simulink model "tire2model"  (R2024b)
settings: Solver=VariableStepAuto  StartTime=0.0  StopTime=20  RelTol=1e-3
PreLoadFcn:
  | Tire = coder.load('Hoosier_R25B_16x75-10x7.mat', 'Tire');
values from neighbouring files (symbols this model uses):
  drive_train_eff = 0.95    [constants.mat]    (also in vehcileConstants2025.m)
  g = 9.81    [constants.mat]    (also in vehcileConstants2025.m)
  i_g = 2.91    [constants.mat]    (also in vehcileConstants2025.m)
  Idx = 1    [ContactPatchLoads.m]    (also in TireEvalModel.m; constants.mat; testing.m; vehcileConstants2025.m)
  Inclination = Inclination   .* (-1).^(mod(Idx+1,2))    [ContactPatchLoads.m]    (also in TireEvalModel.m = params.Inclination; constants.mat = 1; testing.m = 1; vehcileConstants2025.m = 1)
  lr = 0.859026    [constants.mat]    (also in vehcileConstants2025.m)
  m =     [constants.mat]
  Pressure = 70    [ContactPatchLoads.m]    (also in TireEvalModel.m = params.Pressure; constants.mat; testing.m; vehcileConstants2025.m)
  torque_vs_RPM_breakpoints = [0 5500 6048 6500]    [constants.mat]    (also in vehcileConstants2025.m = [0, 5500, 6048, 6500])
  torque_vs_RPM_table = [220 220 170 0]    [constants.mat]    (also in vehcileConstants2025.m = [220, 220, 170, 0])
  wheel =     [constants.mat]
libraries: slpidlib x1, autolibshared x1
settings Model: Creator=nhola  LastModifiedBy=nhola
settings DataIOCC: ExternalInput=[Model Tire]  LoadExternalInput=on
settings DebuggingCC: UnderSpecifiedDimensionMsg=warning

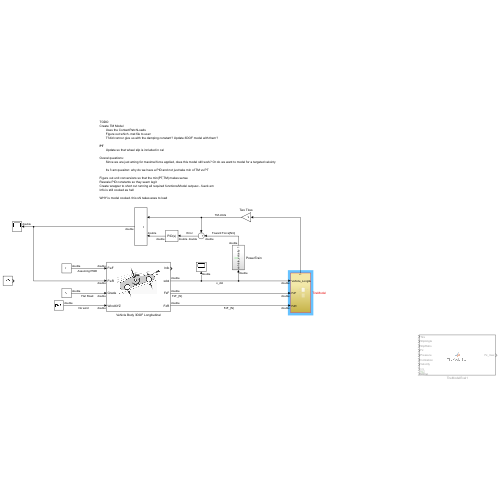
[thumbnail: Simulink's stored preview of the top-level diagram]
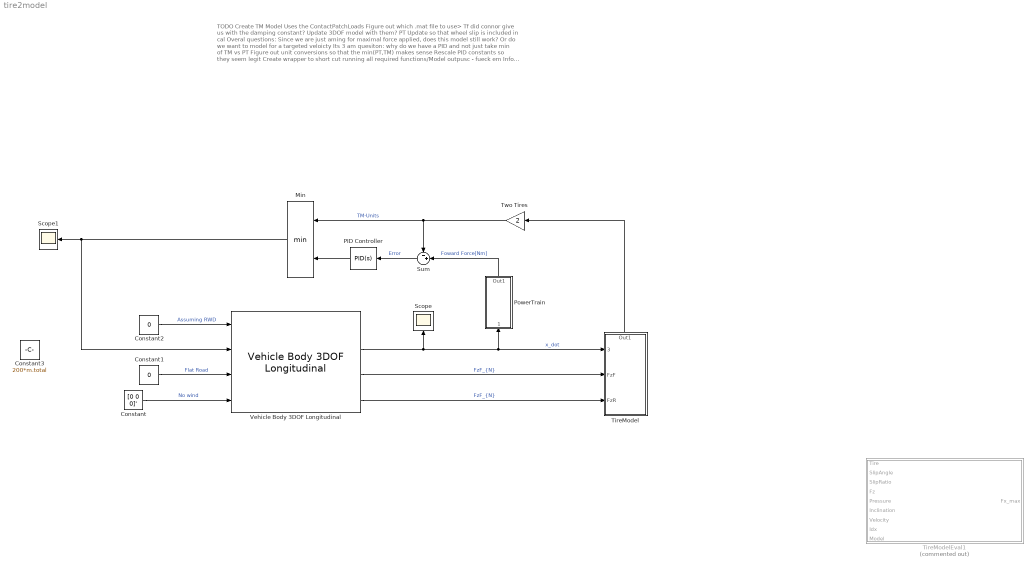
== system tire2model ==
  note: TODO
      | Create TM Model
      | Uses the ContactPatchLoads
      | Figure out which .mat file to use>
      | Tf did connor give us with the damping constant? Update 3DOF model with them?
      |
      | PT
      | Update so that wheel slip is included in cal
      |
      | Overal questions:
      | Since we are just aming for maximal force applied, does this model still work? Or do we want to model for a targeted veloicty
      |
      | Its 3 am quesiton: why do we have a PID and not just take min of TM vs PT
      |
      | Figure out unit conversions so that the min(PT,TM) makes sense
      | Rescale PID constants so they seem legit
      | Create wrapper to short cut running all required functions/Model outpusc - fueck em
      | Info is still cooked as hell
      |
      | WHY is model cooked, this shi takes ages to load
  Constant : Constant  Value=[0 0 0]'  VectorParams1D=off
  Constant1 : Constant  Value=0
  Constant2 : Constant  Value=0
  Constant3 : Constant  Value=200*m.total
  Min : MinMax  Inputs=2
  PID Controller : slpidlib/PID Controller  Controller=PID  Form=Parallel  TimeDomain=Continuous-time  UseExternalTs=off  SampleTime=-1  IntegratorMethod=Forward Euler  FilterMethod=Forward Euler  ControllerParametersSource=internal  P=m.total/5  I=m.total/25  UseKiTs=off  D=m.total/10  UseExternalDerivativeSource=off  N=100  UseFilter=on  TunerSelectOption=Transfer Function Based (PID Tuner App)  InitialConditionSource=internal  InitialConditionForIntegrator=0  InitialConditionForFilter=0  DifferentiatorICPrevScaledInput=0  ExternalReset=none  TrackingMode=off  Kt=1  LimitOutput=off  SatLimitsSource=internal  UpperSaturationLimit=inf  LowerSaturationLimit=-inf  LinearizeAsGain=on  AntiWindupMode=none  Kb=1  LimitIntegrator=off  UpperIntegratorSaturationLimit=inf  LowerIntegratorSaturationLimit=-inf  POutMin=[]  POutMax=[]  IOutMin=[]  IOutMax=[]  DOutMin=[]  DOutMax=[]  NOutMin=[]  NOutMax=[]  SumOutMin=[]  SumOutMax=[]  SaturationOutMin=[]  SaturationOutMax=[]  PParamMin=[]  PParamMax=[]  IParamMin=[]  IParamMax=[]  DParamMin=[]  DParamMax=[]  NParamMin=[]  NParamMax=[]  KbParamMin=[]  KbParamMax=[]  KtParamMin=[]  KtParamMax=[]  KbOutMin=[]  KbOutMax=[]  KtOutMin=[]  KtOutMax=[]  IntegratorOutMin=[]  IntegratorOutMax=[]  FilterOutMin=[]  FilterOutMax=[]  SumI1OutMin=[]  SumI1OutMax=[]  SumI2OutMin=[]  SumI2OutMax=[]  SumI3OutMin=[]  SumI3OutMax=[]  SumI4OutMin=[]  SumI4OutMax=[]  SumDOutMin=[]  SumDOutMax=[]  DifferentiatorOutMin=[]  DifferentiatorOutMax=[]  FilterDiffOutCoefMin=[]  FilterDiffOutCoefMax=[]  ReciprocalOutMin=[]  ReciprocalOutMax=[]  SumDenOutMin=[]  SumDenOutMax=[]  SumNumOutMin=[]  SumNumOutMax=[]  DivideOutMin=[]  DivideOutMax=[]  UdiffTsProdOutMin=[]  UdiffTsProdOutMax=[]  NTsProdOutMin=[]  NTsProdOutMax=[]  UintegralTsProdOutMin=[]  UintegralTsProdOutMax=[]  UngainTsProdOutMin=[]  UngainTsProdOutMax=[]  ClampingZeroOutDataTypeStr=Inherit: Inherit via back propagation  ClampingZeroOutMin=[]  ClampingZeroOutMax=[]  FilterDenConstantOutDataTypeStr=Inherit: Inherit via back propagation  FilterDenConstantOutMin=[]  FilterDenConstantOutMax=[]  PCopyOutDataTypeStr=Inherit: Inherit via back propagation  PCopyOutMin=[]  PCopyOutMax=[]  NCopyOutDataTypeStr=Inherit: Inherit via back propagation  NCopyOutMin=[]  NCopyOutMax=[]  IntegratorContinuousStateAttributes=''  IntegratorStateMustResolveToSignalObject=off  IntegratorRTWStateStorageClass=Auto  FilterContinuousStateAttributes=''  FilterStateMustResolveToSignalObject=off  FilterRTWStateStorageClass=Auto  ParallelPVariant=InternalParameters  IdealPVariant=Disabled  IVariant=InternalParameters  DVariant=InternalParameters  IntegratorVariant=Continuous  SatVariant=Disabled  AWVariant=Passthrough  PCopyVariant=Disabled  TRVariant=Disabled  FdbkBlocksVariant=Forward  IdealPFdbkVariant=Disabled  SatFdbkVariant=Disabled  DerivativeFilterVariant=ContFilter  NVariant=InternalParameters  NCopyVariant=Disabled  FilterICVariant=InternalICsFilter  IntegratorICVariant=InternalICs  ExternalResetVariant=Disabled  TRSumVariant=Passthrough  SumFdbkVariant=Disabled  SumVariant=Sum_PID  TsampFilterVariant=InternalTs  TsampNgainVariant=Passthrough  TsampIntegralVariant=Disabled_SignalSpec  ExternalSaturationOutDataTypeStr=Inherit: Same as second input  DerivativeSourceVariant=ErrorSignal  PreIntVariant=InternalPreInt
  PowerTrain : Subsystem
  Scope : Scope
  Scope1 : Scope
  Sum : Sum  Inputs=-+|
  TireModel : Subsystem
      settings: PortSchema="{\"entries\":[{\"content\":{\"sides\":[{\"content\":{},\"type\":\"ConnectorPlacement.EquallySpacedRectSide\",\"uuid\":\"d4bb879a-aa81-4ea3-92ac-3983b0597440\"},{\"content\":{\"connectorIds\":[\"Out1\"],\"side\":\"RIGHT\"},\"type\":\"ConnectorPlacement.EquallySpacedRectSide\",\"uuid\":\"22ca24d5-9db3-466e-aaa4-c38196519f13\"},{\"content\":{\"connectorIds\":[\"In1\",\"In2\",\"In3\"],\"side\":\"TOP\"},\"type\":\"ConnectorPlacement.EquallySpacedRectSide\",\"uuid\":\"9d20fb85-08e5-4a46-93e2-4c02d14d5f03\"}]},\"type\":\"ConnectorPlacement.EquallySpacedConnector\",\"uuid\":\"57dd96a1-3750-4f3d-ba95-e25498fb6204\"}],\"packageUris\":[\"http://schema.mathworks.com/mf0/Connector/R2020b\"],\"version\":\"1.0\"}"
  TireModelEval1 : MATLAB Function  Commented=on  TreatAsAtomicUnit=on
  Two Tires : Gain  Gain=2
  Vehicle Body 3DOF Longitudinal : autolibshared/Vehicle Body 3DOF Longitudinal  VariantControl=SL  groundType=Grade angle  aMode=2  extFMode=off  extMMode=off  extTamb=off  NF=2  NR=2  m=m.total  a=lf  b=lr  h=hCG  Cd=Cd  Af=A_ref  x_o=0  xdot_o=0  Cl=.1  z_o=-.35  zdot_o=0  Iyy=3500  Cpm=.1  theta_o=0  q_o=0  FskF=[-50, -1, 0, 2, 3, 52].*1.5e4  dzsF=[-5e-3, -1e-4, 0, .2, .2001, .2051]  FsbF=[-10000 -100 -10 0 10 100 10000]  dzdotsF=[-10 -1 -.1 0 .1 1 10]  FskR=[-50, -1, 0, 2, 3, 52].*1e4  dzsR=[-5e-3, -1e-4, 0, .2, .2001, .2051]  FsbR=[-10000 -100 -10 0 10 100 10000]  dzdotsR=[-10 -1 -.1 0 .1 1 10]  Pabs=101325  T=273  g=g  blkID=0
      settings: LibrarySourceBlock=vehdynlibeom/Vehicle Body 3DOF Longitudinal
  wires:
  Constant1/1 -> Vehicle Body 3DOF Longitudinal/3  "Flat Road"
  Constant/1 -> Vehicle Body 3DOF Longitudinal/4  "No wind"
  Constant2/1 -> Vehicle Body 3DOF Longitudinal/1  "Assuming RWD"
  Vehicle Body 3DOF Longitudinal/2 -> Scope/1, PowerTrain/1(vehicle_velocity), TireModel/3(Vehicle_Longitudinal_Velocity)  "x_dot"
  Vehicle Body 3DOF Longitudinal/4 -> TireModel/1(FzR)  "FzF_{N}"
  TireModel/1(Out1) -> Two Tires/1
  Two Tires/1 -> Sum/1, Min/1  "TM-Units"
  Sum/1 -> PID Controller/1  "Error"
  PID Controller/1 -> Min/2
  PowerTrain/1(Out1) -> Sum/2  "Foward Force[Nm]"
  Min/1 -> Vehicle Body 3DOF Longitudinal/2, Scope1/1
  Vehicle Body 3DOF Longitudinal/3 -> TireModel/2(FzF)  "FzF_{N}"

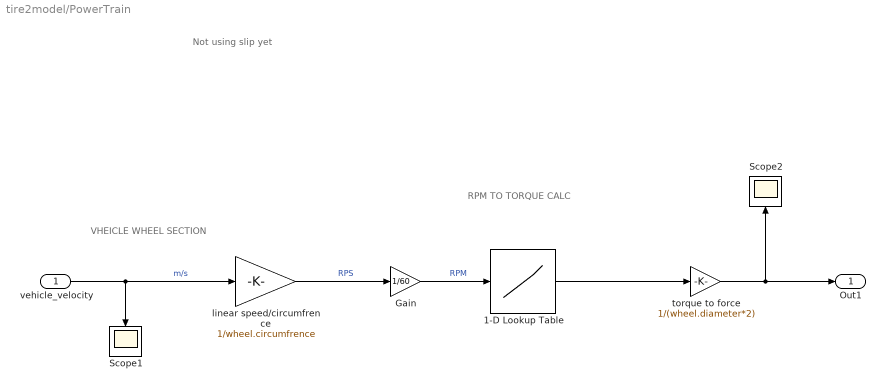
== system tire2model/PowerTrain ==
  note: RPM TO TORQUE CALC
  note: VHEICLE WHEEL SECTION
  note: Not using slip yet
  vehicle_velocity : Inport
  1-D Lookup Table : Lookup_n-D  NumberOfTableDimensions=1  BreakpointsForDimension1=torque_vs_RPM_breakpoints  Table=torque_vs_RPM_table  ExtrapMethod=Clip  UseLastTableValue=on  InternalRulePriority=Speed  RndMeth=Simplest
  Gain : Gain  Gain=1/60
  Scope1 : Scope
  Scope2 : Scope
  linear speed/circumfrence : Gain  Gain=1/wheel.circumfrence
  torque to force : Gain  Gain=1/(wheel.diameter*2)
  Out1 : Outport
  wires:
  vehicle_velocity/1 -> Scope1/1, linear speed/circumfrence/1  "m/s"
  linear speed/circumfrence/1 -> Gain/1  "RPS"
  1-D Lookup Table/1 -> torque to force/1
  torque to force/1 -> Scope2/1, Out1/1
  Gain/1 -> 1-D Lookup Table/1  "RPM"

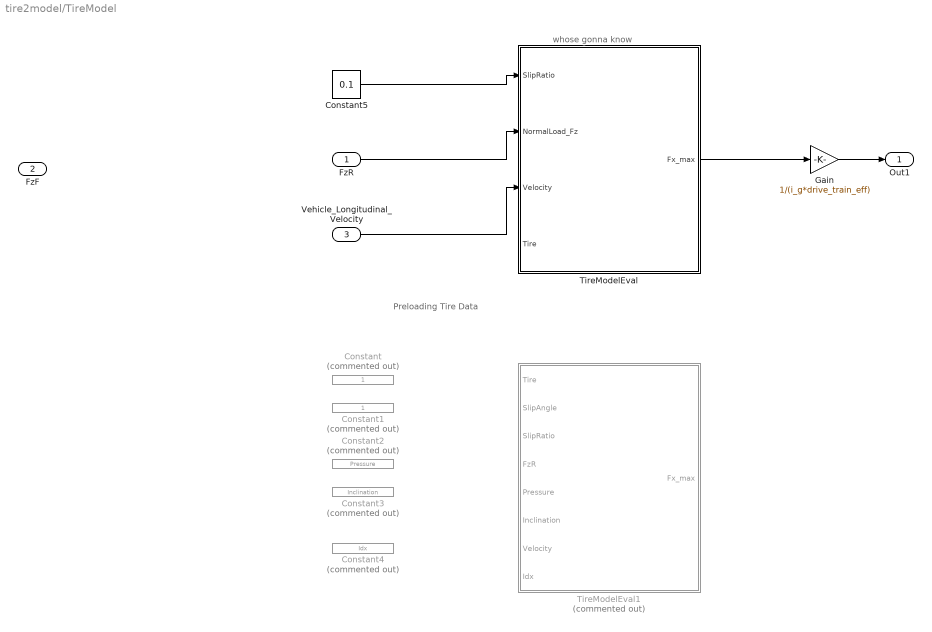
== system tire2model/TireModel ==
  note: Preloading Tire Data
  note: whose gonna know
  FzR : Inport
  FzF : Inport  Port=2
  Vehicle_Longitudinal_Velocity : Inport  Port=3
  Constant : Constant  Commented=on
  Constant1 : Constant  Commented=on
  Constant2 : Constant  Commented=on  Value=Pressure
  Constant3 : Constant  Commented=on  Value=Inclination
  Constant4 : Constant  Commented=on  Value=Idx
  Constant5 : Constant  Value=0.1
  Gain : Gain  Gain=1/(i_g*drive_train_eff)
  TireModelEval : MATLAB Function  TreatAsAtomicUnit=on
  TireModelEval1 : MATLAB Function  Commented=on  TreatAsAtomicUnit=on
  Out1 : Outport
  wires:
  TireModelEval/1(Fx_max) -> Gain/1
  Gain/1 -> Out1/1
  FzR/1 -> TireModelEval/2(NormalLoad_Fz)
  Vehicle_Longitudinal_Velocity/1 -> TireModelEval/3(Velocity)
  Constant5/1 -> TireModelEval/1(SlipRatio)

== matlab function tire2model/TireModel/TireModelEval1 ==
  data: Tire input size=[1 1]; SlipAngle input; SlipRatio input; FzR input; Pressure input; Inclination input; Velocity input; Fx_max output; Idx input
function Fx_max = TireTemp(Tire, SlipAngle, SlipRatio, FzR, Pressure, Inclination, Velocity, Idx)
NormalLoad_Fz=FzR
Model =struct('Pure','Pacejka','Combined','MNC')
% Call the ContactPatchLoads function
[Fx, ~, ~, ~, ~] = ContactPatchLoads(Tire, ...
                                     SlipAngle, ...
                                     SlipRatio, ...
                                     NormalLoad_Fz, ...
                                     Pressure, ...
                                     Inclination, ...
                                     Velocity, ...
                                     Idx, ...
                                     Model);

% Output max longitudinal traction force
Fx_max = Fx;

end

== matlab function tire2model/TireModel/TireModelEval ==
  data: SlipRatio input; NormalLoad_Fz input; Velocity input; Fx_max output; Tire input
function Fx_max = TireModelEval(SlipRatio, NormalLoad_Fz, Velocity, Tire)
%#codegen

% Define static parameters here
Pressure = 70;
Inclination = 1;
Model = 'Pacejka';

% Rest of your code...
dFz = (NormalLoad_Fz - Tire.Pacejka.Fzo) / Tire.Pacejka.Fzo;
dPi = (Pressure - Tire.Pacejka.Pio) / Tire.Pacejka.Pio;
Inc = Inclination;

% Pacejka longitudinal parameters extraction
Cx = Tire.Pacejka.p.C.x(1) .* Tire.Pacejka.L.C.x;
Dx = (Tire.Pacejka.p.D.x(1) + Tire.Pacejka.p.D.x(2)*dFz) .* ...
     (1 - Tire.Pacejka.p.D.x(3)*Inc^2).*NormalLoad_Fz.*Tire.Pacejka.L.mu.x;

Ex = ( Tire.Pacejka.p.E.x(1) + Tire.Pacejka.p.E.x(2)*dFz ...
    + Tire.Pacejka.p.E.x(3)*dFz^2 ) .* ( 1 - Tire.Pacejka.p.E.x(4)*sign(SlipRatio) ) ...
    .* Tire.Pacejka.L.E.x;

Kxk = NormalLoad_Fz.*(Tire.Pacejka.p.K.x(1) + Tire.Pacejka.p.K.x(2)*dFz ) .* ...
      exp( Tire.Pacejka.p.K.x(3) .* dFz ) .* Tire.Pacejka.L.K.x.k;

Bx = Kxk ./ ( Cx.*Dx );
Vx = NormalLoad_Fz.*(Tire.Pacejka.p.V.x(1) + Tire.Pacejka.p.V.x(2)*dFz ) .* ...
      Tire.Pacejka.L.V.x;
Hx = (Tire.Pacejka.p.H.x(1) + Tire.Pacejka.p.H.x(2)*dFz) .* Tire.Pacejka.L.H.x;

% Compute Pacejka Longitudinal Force (Fx)
Fx_max = Dx .* sin( Cx .* atan( (1-Ex) .* Bx.*(SlipRatio + Hx) + ...
             Ex .* atan( Bx.*(SlipRatio + Hx) ) ) ) + Vx;
end

== matlab function tire2model/TireModelEval1 ==
  data: Tire input; SlipAngle input size=[1 1]; SlipRatio input; Fz input; Pressure input; Inclination input; Velocity input; Fx_max output size=[1 1]; Idx input; Model input
function Fx_max = TireModelEval(Tire, SlipAngle, SlipRatio, Fz, Pressure, Inclination, Velocity, Idx, Model)


    SlipAngle = 0; % Straight-line acceleration
    [Fx, ~, ~, ~, ~] = ContactPatchLoads(Tire, SlipAngle, SlipRatio, Fz, Pressure, Inclination, Velocity, Idx, Model);
    
    % Output maximum allowable Fx based on slip
    Fx_max = Fx;


end
